simulink model "PVModelPSO"  (R2020a)
settings: Solver=VariableStepAuto  StartTime=0.0  StopTime=2  MaxStep=1e-4  RelTol=1e-3
libraries: powerlib x17, re_lib x5, powerlib_meascontrol x1
settings Model: Creator=Mahesh Krishna  LastModifiedBy=user
settings DataIOCC: ReturnWorkspaceOutputs=off
settings OptimizationCC: LifeSpan=inf
settings DebuggingCC: ArithmeticOperatorsInVariantConditions=warning
settings SFSimCC: SimUseLocalCustomCode=off  CustomCodeUndefinedFunction=UseInterfaceOnly
settings RTWCC: RTWUseLocalCustomCode=off
settings CodeAppCC: StateflowObjectComments=on
settings SimscapeCC: SimscapeNormalizeSystem=off

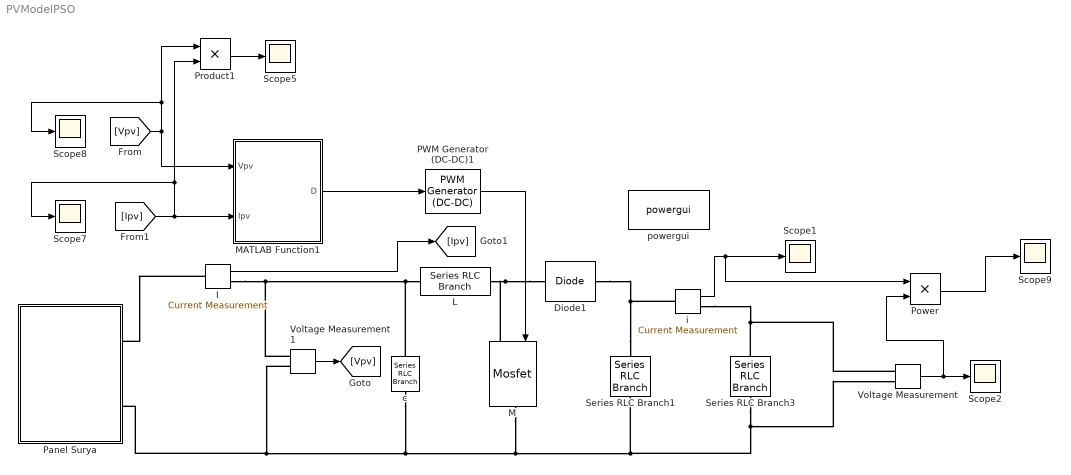
== system PVModelPSO ==
  Diode1 : powerlib/Power Electronics/Diode  Ron=1e-3  Lon=0  Vf=0  IC=0  UseSnubber=off  Rs=inf  Cs=inf  Measurements=off
  I : powerlib/Measurements/Current Measurement  PhasorSimulation=off  OutputType=Magnitude  PSBequivalent=0
  L : powerlib/Elements/Series RLC Branch  LConnTagsString=__new0  RConnTagsString=__new0  BranchType=L  Resistance=1e-3  Inductance=5e-3  SetiL0=off  InitialCurrent=0  Capacitance=1e-6  Setx0=off  InitialVoltage=0  Measurements=None
  M : powerlib/Power Electronics/Mosfet  Ron=1e-3  Lon=0  Rd=1e-3  Vfd=0  IC=0  Rs=inf  Cs=inf  Measurements=off
  MATLAB Function1 : MATLAB Function  TreatAsAtomicUnit=on
  PWM Generator (DC-DC)1 : powerlib_meascontrol/Pulse & Signal Generators/PWM Generator (DC-DC)  Fsw=20000  Ts=0
  Panel Surya : Subsystem
  Power : Product
  Product1 : Product
  Scope{1..2,5,7..9} (6 alike) : Scope
  Series RLC Branch1 : powerlib/Elements/Series RLC Branch  LConnTagsString=__new0  RConnTagsString=__new0  BranchType=C  Resistance=1e-4  Inductance=200e-6  SetiL0=off  InitialCurrent=0  Capacitance=22e-6  Setx0=off  InitialVoltage=40  Measurements=None
  Series RLC Branch3 : powerlib/Elements/Series RLC Branch  LConnTagsString=__new0  RConnTagsString=__new0  BranchType=R  Resistance=100  Inductance=200e-6  SetiL0=off  InitialCurrent=0  Capacitance=1000e-6  Setx0=off  InitialVoltage=40  Measurements=None
  Voltage Measurement : powerlib/Measurements/Voltage Measurement  PhasorSimulation=off  OutputType=Magnitude  PSBequivalent=0
  Voltage Measurement1 : powerlib/Measurements/Voltage Measurement  PhasorSimulation=off  OutputType=Magnitude  PSBequivalent=0
  c : powerlib/Elements/Series RLC Branch  LConnTagsString=__new0  RConnTagsString=__new0  BranchType=C  Resistance=1e-3  Inductance=250e-6  SetiL0=off  InitialCurrent=0  Capacitance=2.2e-6  Setx0=off  InitialVoltage=0  Measurements=None
  i : powerlib/Measurements/Current Measurement  PhasorSimulation=off  OutputType=Magnitude  PSBequivalent=0
  powergui : powerlib/powergui  Priority=1  SimulationMode=Continuous  SampleTime=50e-6  frequency=60  Iterations=50  frequencyindice=0  Pbase=100e6  ErrMax=1e-4  UnitsV=kV  UnitsW=MW  buscounter=0  FunctionMessages=off  echomessages=off  EnableUseOfTLC=off  CurrentSourceSwitches=off  DisableSnubberDevices=off  DisableRonSwitches=off  DisableVfSwitches=off  DisplayEquations=off  AutomaticDiscreteSolvers=off  SolverType=Tustin/Backward Euler (TBE)  Interpol=off  ExternalGateDelay=off  methode=off  Ts=100  x0status=blocks  SPID=on  SwTol=0  HookPort=off  NonlinearTolerance=1e-4  nMaxIteration=100  ContinueOnMaxIteration=off  RestoreLinks=warning  ResistiveCurrentMeasurement=off  Frange=[0:2:500]  Ylog=off  Xlog=on  ShowGrid=off  save=off  variable=ZData  structure=0  ZoomFFT=off  StartTime=0.0  cycles=1  DisplayStyle=1  fundamental=60  FreqAxis=off  MaxFrequency=1000  frequencyindicesteady=1  RmsSteady=1  display=off
  wires:
  I/1 -> [Ipv]
  [Ipv] -> Scope7/1, Product1/2, MATLAB Function1/2(Ipv)
  Voltage Measurement/1 -> Power/2, Scope2/1
  PWM Generator (DC-DC)1/1 -> M/1
  i/1 -> Power/1, Scope1/1
  Voltage Measurement1/1 -> [Vpv]
  [Vpv] -> MATLAB Function1/1(Vpv), Scope8/1, Product1/1
  Product1/1 -> Scope5/1
  Power/1 -> Scope9/1
  MATLAB Function1/1(D) -> PWM Generator (DC-DC)1/1
  connections:
  i/RConn1 -- Series RLC Branch3/LConn1 -- Voltage Measurement/LConn1
  Series RLC Branch1/RConn1 -- Series RLC Branch3/RConn1 -- Voltage Measurement/LConn2 -- Voltage Measurement1/LConn2 -- Panel Surya/RConn2 -- c/RConn1 -- M/RConn1
  Series RLC Branch1/LConn1 -- Diode1/RConn1 -- i/LConn1
  I/LConn1 -- Panel Surya/RConn1
  Diode1/LConn1 -- M/LConn1 -- L/RConn1
  I/RConn1 -- Voltage Measurement1/LConn1 -- c/LConn1 -- L/LConn1

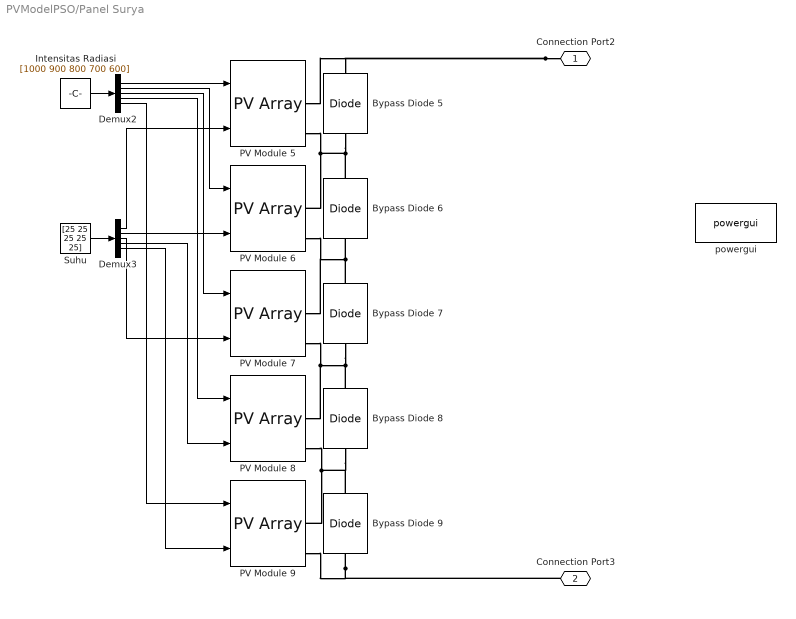
== system PVModelPSO/Panel Surya ==
  Bypass Diode {5..9} (5 alike) : powerlib/Power Electronics/Diode  Ron=0.001  Lon=0  Vf=0.8  IC=0  UseSnubber=off  Rs=500  Cs=250e-9  Measurements=off
  Demux2 : Demux  Outputs=5
  Demux3 : Demux  Outputs=5
  Intensitas Radiasi : Constant  Value=[1000 900 800 700 600]
  PV Module {5..9} (5 alike) : re_lib/Solar/PV Array  Npar=1  Nser=1  PlotType=array @ 1000 W/m2 & specified temperatures  S_vec="[ 1000  500  100 ]"  Temp_C_vec="[ 45 25  ]"  ModuleName=ET Solar Industry ET-P654200WW  PlotWhenSelected=off  Pm=200.2656  Ncell=54  Voc=32.72  Isc=7.86  Vm=27.21  Im=7.36  beta_Voc_pc=-0.35691  alpha_Isc_pc=0.050102  beta_Voc=-0.11678  alpha_Isc=0.003938  IL=7.8912  I0=2.3497e-10  nI=0.974  Rsh=176.8846  Rs=0.19523  RobustModel=off  RobustCellTemperature=25  BAL=off  Tc=1e-6  Tfilter=5e-5
  Suhu : Constant  Value=[25 25 25 25 25]
  powergui : powerlib/powergui  Priority=1  SimulationMode=Continuous  SampleTime=50e-6  frequency=60  Iterations=50  frequencyindice=0  Pbase=100e6  ErrMax=1e-4  UnitsV=kV  UnitsW=MW  buscounter=0  FunctionMessages=off  echomessages=off  EnableUseOfTLC=off  CurrentSourceSwitches=off  DisableSnubberDevices=off  DisableRonSwitches=off  DisableVfSwitches=off  DisplayEquations=off  AutomaticDiscreteSolvers=off  SolverType=Tustin/Backward Euler (TBE)  Interpol=off  ExternalGateDelay=off  methode=off  Ts=100  x0status=blocks  SPID=on  SwTol=0  HookPort=off  NonlinearTolerance=1e-4  nMaxIteration=100  ContinueOnMaxIteration=off  RestoreLinks=warning  ResistiveCurrentMeasurement=off  Frange=[0:2:500]  Ylog=off  Xlog=on  ShowGrid=off  save=off  variable=ZData  structure=0  ZoomFFT=off  StartTime=0.0  cycles=1  DisplayStyle=1  fundamental=60  FreqAxis=off  MaxFrequency=1000  frequencyindicesteady=1  RmsSteady=1  display=off
  Connection Port2 : PMIOPort  Side=Right
  Connection Port3 : PMIOPort  Port=2  Side=Right
  wires:
  Demux2/1 -> PV Module 5/1
  Demux3/4 -> PV Module 8/2
  Demux3/1 -> PV Module 5/2
  Demux3/3 -> PV Module 7/2
  Demux2/5 -> PV Module 9/1
  Demux2/4 -> PV Module 8/1
  Demux2/3 -> PV Module 7/1
  Demux3/5 -> PV Module 9/2
  Intensitas Radiasi/1 -> Demux2/1
  Demux2/2 -> PV Module 6/1
  Suhu/1 -> Demux3/1
  Demux3/2 -> PV Module 6/2
  connections:
  Bypass Diode 6/RConn1 -- Bypass Diode 5/LConn1 -- PV Module 5/RConn2 -- PV Module 6/RConn1
  Connection Port2/RConn1 -- PV Module 5/RConn1 -- Bypass Diode 5/RConn1
  Bypass Diode 9/LConn1 -- Connection Port3/RConn1 -- PV Module 9/RConn2
  Bypass Diode 7/RConn1 -- Bypass Diode 6/LConn1 -- PV Module 7/RConn1 -- PV Module 6/RConn2
  PV Module 8/RConn2 -- PV Module 9/RConn1 -- Bypass Diode 8/LConn1 -- Bypass Diode 9/RConn1
  PV Module 7/RConn2 -- PV Module 8/RConn1 -- Bypass Diode 7/LConn1 -- Bypass Diode 8/RConn1

== matlab function PVModelPSO/MATLAB Function1 ==
  settings: updateMethod=DISCRETE  sampleTime=1e-4
  data: Vpv input; D output; Ipv input
function D = PSO(Vpv,Ipv)
coder.extrinsic('rand')
%% inisialisasi parameter dan deklarasi variabel persistent
persistent iterasi cekpartikel counter counter2 kecepatan posisi fitness fitnessPbest Pbest fitnessGbest Gbest cekKonvergen cekBerhenti berhenti Gbestakhir;

partikel = 5;
maxiterasi = 30;

%batas bawah dan batas atas posisi
dmin = 0;
dmax = 0.95;

% nilai w c1 dan c2
w=0.4;
c1=1;
c2=1.6;

%batas bawah dan batas atas kecepatan
vmax =0.6*((dmax-dmin)/2);
vmin = -1*vmax;

%nilai toleransi untuk konvergen
toleransi = 5;

%nilai random untuk inisialisasi posisi
r1 = zeros(partikel,1);
r1 = rand(partikel,1);


%nilai random untuk update kecepatan
r2 = zeros(maxiterasi*partikel,1);
r3 = zeros(maxiterasi*partikel,1);

r2 = rand(maxiterasi*partikel,1);
r3 = rand(maxiterasi*partikel,1);

%% inisialisasi variabel setelah dideklarasikan    
if(isempty(iterasi))
    iterasi=1;
end

if(isempty(cekpartikel))
    cekpartikel = 1;
end

if(isempty(counter))
    counter=1;
end

if(isempty(counter2))
    counter2=1;
end

%inisialisasi posisi
if(isempty(posisi))
    posisi = zeros(partikel,1);
    for i=1:partikel
        posisi(i)=dmin+r1(i)*(dmax-dmin);
    end
end

%inisialisasi kecepatan
if(isempty(kecepatan))
    kecepatan = zeros(partikel,1);
end

if(isempty(fitness))
    fitness = zeros(partikel,1);
end

if(isempty(fitnessPbest))
    fitnessPbest = zeros(partikel,1);
end

if(isempty(Pbest))
    Pbest = zeros(partikel,1);
end

if(isempty(Gbest))
    Gbest = zeros(maxiterasi,1);
end

if(isempty(fitnessGbest))
    fitnessGbest = zeros(maxiterasi,1);
end

if(isempty(cekKonvergen))
    cekKonvergen = zeros(5,1);
end

if(isempty(cekBerhenti))
    cekBerhenti = zeros(5,1);
end

if(isempty(berhenti))
    berhenti = 0;
end

if(isempty(Gbestakhir))
    Gbestakhir = 0;
end
%% evaluasi duty cycle
%duty cycle dievaluasi hingga 200 kali hingga mendapat nilai yang stabil
if(counter>=1 && counter<=200)
    D=posisi(cekpartikel);
    counter=counter+1;
    if(berhenti==1)
        D=Gbestakhir;
        counter=counter-1;
    end
    return;
else
    if(cekpartikel<=4)
        D=posisi(cekpartikel+1);
    else
        D=posisi(1);
    end
end
%% Main  PSO
fitness(cekpartikel) = Vpv*Ipv;
%loop partikel dalam iterasi
if(cekpartikel<=4)
    cekpartikel = cekpartikel+1;
    counter = 2; %setelah dilakukan evaluasi duty cycle, nilai counter dikembalikan untuk evaluasi duty cycle partikel selanjutnya
else
    if(iterasi==1)
        %inisialisasi Pbest
        for i=1:partikel
            Pbest(i) = posisi(i);
            fitnessPbest(i) = fitness(i);
        end
        maxFitnessPbest = 0;
        for j = 1:length(fitnessPbest)
            if fitnessPbest(j) > maxFitnessPbest
                maxFitnessPbest = fitnessPbest(j);
            end
        end
        fitnessGbest(iterasi) = maxFitnessPbest;
        for k=1:partikel
            if(fitnessGbest(iterasi) == fitnessPbest(k))
                Gbest(iterasi) = Pbest(k);
            end
        end
    elseif(iterasi >=2 && iterasi<=maxiterasi)
        %update Pbest
        for i=1:partikel
            if (fitness(i) > fitnessPbest(i))
                Pbest(i) = posisi(i);
                fitnessPbest(i) = fitness(i);
            end
        end
        %update Gbest
        maxFitnessPbest = 0;
        for j = 1:length(fitnessPbest)
            if fitnessPbest(j) > maxFitnessPbest
                maxFitnessPbest = fitnessPbest(j);
            end
        end
        fitnessGbest(iterasi) = maxFitnessPbest;
        for k=1:partikel
            if(fitnessGbest(iterasi) == fitnessPbest(k))
                Gbest(iterasi) = Pbest(k);
            end
        end
    end
    %cek konvergen setiap partikel
    for i=1:partikel
        if ((fitnessGbest(iterasi) - fitnessPbest(i)) < toleransi)
            cekBerhenti(i)=1;
        end
    end
    n = sum(cekBerhenti);
    %jika semua partikel sudah konvergen
    if(n==5)
        berhenti = 1;
        Gbestakhir = Gbest(iterasi);
    else
        cekBerhenti = zeros(partikel,1);
    end
    %update kecepatan dan posisi
    for i=1:partikel
        %update kecepatan
        kecepatan(i) = (w*kecepatan(i))+(c1*r2(counter2)*(Pbest(i)-posisi(i)))+(c2*r3(counter2)*(Gbest(iterasi)-posisi(i)));
        counter2 = counter2+1;
        %perbaikan update kecepatan
        if(kecepatan(i) > vmax)
            kecepatan(i)=vmax;
        end
        if(kecepatan(i)<vmin)
            kecepatan(i)=vmin;
        end
        
        %update posisi
        posisi(i) = posisi(i) + kecepatan(i);
        %perbaikan update posisi
        if(posisi(i) > dmax)
            posisi(i)=dmax;
        end
        if(posisi(i)<dmin)
            posisi(i)=dmin;
        end
    end
    D=posisi(1);
    cekpartikel = 1;
    counter = 2; %setelah dilakukan evaluasi duty cycle, nilai counter dikembalikan untuk evaluasi duty cycle partikel selanjutnya
    iterasi = iterasi+1;
end
end
